simulink model "ES3011_Lab4_Q4"  (R2023b)
settings: Solver=VariableStepAuto  StartTime=0.0  StopTime=10.0  RelTol=1e-3
values from neighbouring files (symbols this model uses):
  b = 20    [q1.m]    (also in q2.m = 50; q2_tuning.m = 50; q3.m = 3.51e-06; q4.m = 50)
  Ki = 1    [q2_2.m]    (also in q2_tuning.m; q4.m = 40)
  Kp = 100    [q2_2.m]    (also in q2_tuning.m; q4.m = 800)
  m = 1    [q1.m]    (also in q2.m = 1500; q2_tuning.m = 1500; q4.m = 1500)
settings Model: Creator=cap1sup  LastModifiedBy=cap1sup

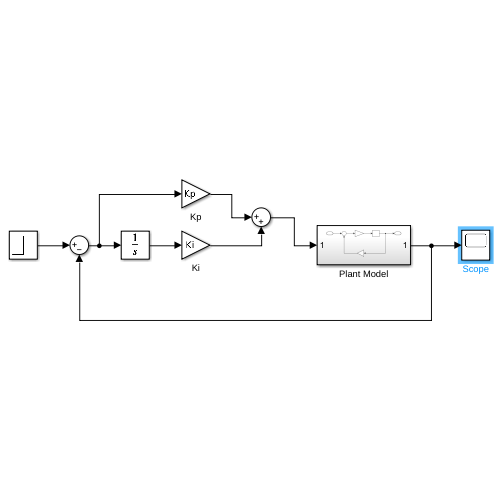
[thumbnail: Simulink's stored preview of the top-level diagram]
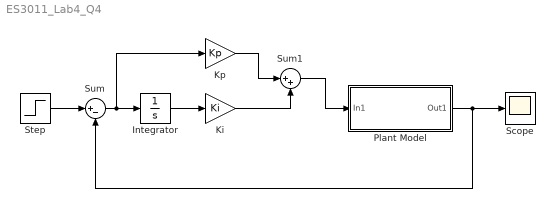
== system ES3011_Lab4_Q4 ==
  Integrator : Integrator
  Ki : Gain  Gain=Ki
  Kp : Gain  Gain=Kp
  Plant Model : Subsystem
  Scope : Scope
  Step : Step  Time=0  After=u  SampleTime=0
  Sum : Sum  Inputs=|+-
  Sum1 : Sum  Inputs=|++
  wires:
  Plant Model/1(Out1) -> Scope/1, Sum/2
  Sum/1 -> Kp/1, Integrator/1
  Integrator/1 -> Ki/1
  Kp/1 -> Sum1/1
  Ki/1 -> Sum1/2
  Sum1/1 -> Plant Model/1(In1)
  Step/1 -> Sum/1

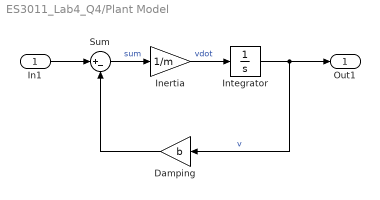
== system ES3011_Lab4_Q4/Plant Model ==
  In1 : Inport
  Damping : Gain  Gain=b
  Inertia : Gain  Gain=1/m
  Integrator : Integrator
  Sum : Sum  Inputs=|+-
  Out1 : Outport
  wires:
  Damping/1 -> Sum/2
  In1/1 -> Sum/1
  Integrator/1 -> Out1/1, Damping/1  "v"
  Inertia/1 -> Integrator/1  "vdot"
  Sum/1 -> Inertia/1  "sum"
